simulink model "ChiefMaster_TTC580"  (R2022b)
settings: Solver=FixedStepAuto  StartTime=0.0  StopTime=10  FixedStep=0.01  RelTol=1e-3
values from neighbouring files (symbols this model uses):
  BattBox1_No = single(1)    [Parameters.m]
  BattBox2_No = single(2)    [Parameters.m]
  BattBox3_No = single(3)    [Parameters.m]
  CurrentLB = single(-3)    [Parameters.m]
  CurrentReductionConstant_Lvl0 = single(0.03)    [Parameters.m]
  CurrentReductionConstant_Lvl1 = single(0.05)    [Parameters.m]
  CurrentReductionConstant_Lvl2 = single(0.07)    [Parameters.m]
  CurrentReductionConstant_Lvl3 = single(0.1)    [Parameters.m]
  CurrentUB = single(3)    [Parameters.m]
  DCHV_Minus_In_Delay_ms = single(500)    [Parameters.m]
  FL_sHVC_CellBalanceVoltage_mV = single(3500)    [Parameters.m]
  FL_sInrushCurrent_dividebyzero = single(0.00001)    [Parameters.m]
  FL_u8HMI_BuzzerTimer = uint8(3)    [Parameters.m]
  IP_boActValue = true    [Parameters.m]
  IP_boDeactValue = false    [Parameters.m]
  IP_boInitValue = false    [Parameters.m]
  IP_s_LB = 18000    [Parameters.m]
  IP_s_UB = 22000    [Parameters.m]
  IP_sBatt1_ChargeCurrentMax_Factor = single(0.1)    [Parameters.m]
  IP_sBatt1_ChargeCurrentMax_LB = single(0)    [Parameters.m]
  IP_sBatt1_ChargeCurrentMax_Offset = single(0)    [Parameters.m]
  IP_sBatt1_ChargeCurrentMax_UB = single(6553.5)    [Parameters.m]
  IP_sBatt1_Current_Factor = single(0.1)    [Parameters.m]
  IP_sBatt1_Current_LB = single(-3276.8)    [Parameters.m]
  IP_sBatt1_Current_Offset = single(0)    [Parameters.m]
  IP_sBatt1_Current_UB = single(3276.8)    [Parameters.m]
  IP_sBatt1_DisChargeCurrentMax_Factor = single(0.1)    [Parameters.m]
  IP_sBatt1_DisChargeCurrentMax_LB = single(0)    [Parameters.m]
  IP_sBatt1_DisChargeCurrentMax_Offset = single(0)    [Parameters.m]
  IP_sBatt1_DisChargeCurrentMax_UB = single(6553.5)    [Parameters.m]
  IP_sBatt1_InsulationResistance_Factor = single(5)    [Parameters.m]
  IP_sBatt1_InsulationResistance_LB = single(0)    [Parameters.m]
  IP_sBatt1_InsulationResistance_Offset = single(0)    [Parameters.m]
  IP_sBatt1_InsulationResistance_UB = single(0)    [Parameters.m]
  IP_sBatt1_LiBa_IntResist_mOhm = single(25)    [Parameters.m]
  IP_sBatt1_SOC_Factor = single(1)    [Parameters.m]
  IP_sBatt1_SOC_LB = single(0)    [Parameters.m]
  IP_sBatt1_SOC_Offset = single(0)    [Parameters.m]
  IP_sBatt1_SOC_UB = single(100)    [Parameters.m]
  IP_sBatt1_SOH_Factor = single(1)    [Parameters.m]
  IP_sBatt1_SOH_LB = single(0)    [Parameters.m]
  IP_sBatt1_SOH_Offset = single(0)    [Parameters.m]
  IP_sBatt1_SOH_UB = single(100)    [Parameters.m]
  IP_sBatt1_Ubatt_Factor = single(0.1)    [Parameters.m]
  IP_sBatt1_Ubatt_LB = single(0)    [Parameters.m]
  IP_sBatt1_Ubatt_Offset = single(0)    [Parameters.m]
  IP_sBatt1_Ubatt_UB = single(6553.5)    [Parameters.m]
  IP_sBatt1_UserRi_Factor = single(1)    [Parameters.m]
  IP_sBatt1_UserRi_LB = single(0)    [Parameters.m]
  IP_sBatt1_UserRi_Offset = single(0)    [Parameters.m]
  IP_sBatt1_UserRi_UB = single(255)    [Parameters.m]
  IP_sBatt1_VoltageAtSensor_Factor = single(0.02)    [Parameters.m]
  IP_sBatt1_VoltageAtSensor_LB = single(0)    [Parameters.m]
  IP_sBatt1_VoltageAtSensor_Offset = single(0)    [Parameters.m]
  IP_sBatt1_VoltageAtSensor_UB = single(1310.7)    [Parameters.m]
  IP_sBatt2_LiBa_IntResist_mOhm = single(25)    [Parameters.m]
  IP_sBatt3_LiBa_IntResist_mOhm = single(25)    [Parameters.m]
  IP_sEM_LB = 2000    [Parameters.m]
  IP_sEM_UB = 8000    [Parameters.m]
  IP_sFB_LB = 5000    [Parameters.m]
  IP_sFB_UB = 10000    [Parameters.m]
  IP_sHVIL_LB = 12000    [Parameters.m]
  IP_sHVIL_UB = 15000    [Parameters.m]
  IP_sLoad_Voltage_Factor = single(1)    [Parameters.m]
  IP_sLoad_Voltage_LB = single(0)    [Parameters.m]
  IP_sLoad_Voltage_Offset = single(0)    [Parameters.m]
  IP_sLoad_Voltage_UB = single(65535)    [Parameters.m]
  IP_u8HVIL_Delay_ms = uint8(100)    [Parameters.m]
  IP_u8HW_IN_delay_ms = uint8(100)    [Parameters.m]
  IT_sInsulationSafeValue_kOhm = single(650)    [Parameters.m]
  IT_u8IMD_DelayTime_s = uint8(20)    [Parameters.m]
  MainHV_Minus_In_Delay = single(5)    [Parameters.m]
  MainHV_StatusDelay = single(5)    [Parameters.m]
  NotAvailable_uint16 = single(65535)    [Parameters.m]
  NotAvailable_uint8 = uint8(255)    [Parameters.m]
  OP_boHVIL_Supply = boolean(1)    [Parameters.m]
  SafeCurrentToCloseHV_A = single(5)    [Parameters.m]
  SafeVoltageToCloseHV_V = single(0.5)    [Parameters.m]
  UnexpectedBattChargingFcn_Available = boolean(1)    [Parameters.m]
  Voltage_NA_UB = uint16(65535)    [Parameters.m]
  VoltageSensorAvailableBB1 = boolean(0)    [Parameters.m]
  VoltageSensorAvailableBB2 = boolean(0)    [Parameters.m]
  VoltageSensorAvailableBB3 = boolean(0)    [Parameters.m]
libraries: simulink x184, Library_DataProcessing_v1_1 x167, Library_DataProcessing_v1 x142, libCM x28
(part 1 of 19)
settings Model: TunableVars=SafeCurrentToCloseHV_A,SafeVoltageToCloseHV_V,Voltage_NA_UB,MainHV_Minus_In_Delay,MainHV_StatusDelay,BattBox1_No,BattBox2_No,BattBox3_No,NotAvailable_uint16,NotAvailable_uint8,VoltageSensorAvailableBB1,VoltageSensorAvailableBB2,VoltageSensorAvailableBB3,CurrentLB,CurrentReductionConstant_Lvl0,CurrentReductionConstant_Lvl1,CurrentReductionConstant_Lvl2,CurrentReductionConstant_Lvl3,CurrentUB,FL_sHVC_CellBalanceVoltage_mV,FL_sInrushCurrent_dividebyzero,FL_u8HMI_BuzzerTimer,UnexpectedBattChargingFcn_Available,IT_sInsulationSafeValue_kOhm,DCHV_Minus_In_Delay_ms,IP_u8HW_IN_delay_ms,OP_boHVIL_Supply,IP_u8HVIL_Delay_ms,IT_u8IMD_DelayTime_s  TunableVarsStorageClass=ExportedGlobal,ExportedGlobal,ExportedGlobal,ExportedGlobal,ExportedGlobal,ExportedGlobal,ExportedGlobal,ExportedGlobal,ExportedGlobal,ExportedGlobal,ExportedGlobal,ExportedGlobal,ExportedGlobal,ExportedGlobal,ExportedGlobal,ExportedGlobal,ExportedGlobal,ExportedGlobal,ExportedGlobal,ExportedGlobal,ExportedGlobal,ExportedGlobal,ExportedGlobal,ExportedGlobal,ExportedGlobal,ExportedGlobal,ExportedGlobal,ExportedGlobal,ExportedGlobal  TunableVarsTypeQualifier=,,,,,,,,,,,,,,,,,,,,,,,,,,,,  Creator=SidharthUrbanMobilit  LastModifiedBy=NurdoganUrbanMobilit
settings SolverCC: AlgebraicLoopSolver=TrustRegion
settings OptimizationCC: DefaultUnderspecifiedDataType=single  ZeroExternalMemoryAtStartup=off  ZeroInternalMemoryAtStartup=off  NoFixptDivByZeroProtection=on  EfficientFloat2IntCast=on  EfficientTunableParamExpr=on
settings DebuggingCC: SignalInfNanChecking=error  ParameterPrecisionLossMsg=none  ParameterTunabilityLossMsg=error  UnconnectedInputMsg=warning  UnconnectedOutputMsg=warning  UnconnectedLineMsg=warning  FrameProcessingCompatibilityMsg=none  BusObjectLabelMismatch=error  SFMachineParentedDataDiag=warning
settings ModelReferenceCC: EnableRefExpFcnMdlSchedulingChecks=on
settings SFSimCC: MATLABDynamicMemAlloc=off
settings RTWCC: Description=Embedded Coder  SystemTargetFile=ert.tlc  TemplateMakefile=ert_default_tmf  DLArmComputeVersion=19.05
settings CodeAppCC: ForceParamTrailComments=on  MaxIdLength=100  OperatorAnnotations=on  SimulinkDataObjDesc=on  SFDataObjDesc=on  MATLABFcnDesc=on  CustomSymbolStrFcn=$N$M  CustomSymbolStrFcnArg=$N$M  InsertBlockDesc=on  StateflowObjectComments=on  MATLABSourceComments=on  ReqsInCode=on
settings ERTTargetCC: TargetLangStandard=C99 (ISO)  CodeReplacementLibrary=PLC  GenerateSampleERTMain=on  SupportNonFinite=off  SupportVariableSizeSignals=on  ERTCustomFileTemplate=example_file_process.tlc
settings ConfigComp: PLC_OutputDir=cdsys  PLC_TargetIDE=codesys35  PLC_MultiTBSigbuilderTimeRange=off  PLC_PreserveAliasType=on  PLC_FoldFBCallOutputVar=off  PLC_OverrideDefaultNameLength=on  PLC_InlineEnumCastFunction=off  PLC_RTWMaxIdLength=100  PLC_GenerateReport=off  PLC_LaunchReport=off

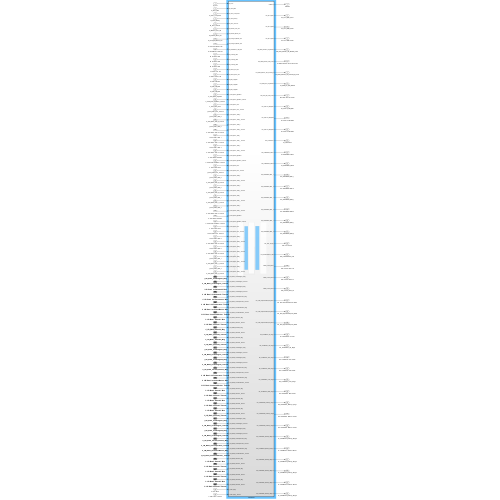
[thumbnail: Simulink's stored preview of the top-level diagram]
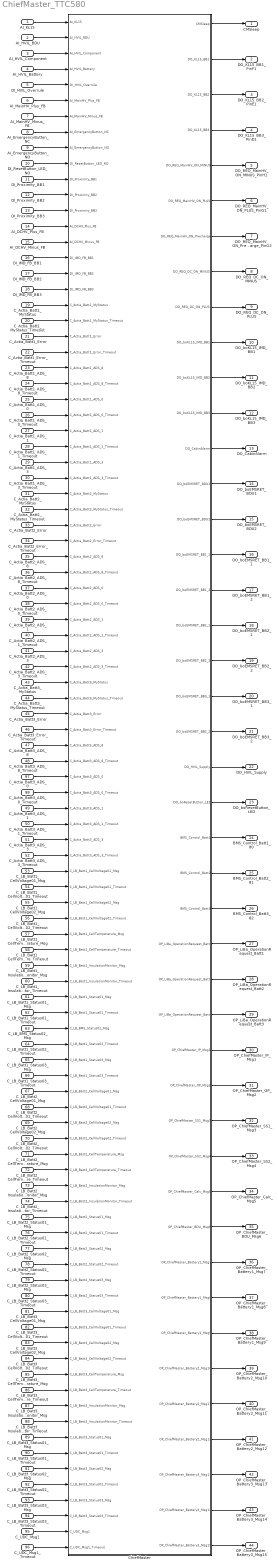
== system ChiefMaster_TTC580 ==
  AI_KL15 : Inport  OutDataTypeStr=single
  AI_HVIL_BDU : Inport  Port=2  OutDataTypeStr=single
  AI_HVIL_Component : Inport  Port=3  OutDataTypeStr=single
  AI_HVIL_Battery : Inport  Port=4  OutDataTypeStr=single
  DI_HVIL_Overrule : Inport  Port=5  OutDataTypeStr=boolean
  AI_MainHV_Plus_FB : Inport  Port=6  OutDataTypeStr=single
  AI_MainHV_Minus_FB : Inport  Port=7  OutDataTypeStr=single
  AI_EmergencyButton_NC : Inport  Port=8  OutDataTypeStr=single
  AI_EmergencyButton_NO : Inport  Port=9  OutDataTypeStr=single
  DI_ResetButton_LED_NO : Inport  Port=10  OutDataTypeStr=boolean
  DI_Proximity_BB1 : Inport  Port=11  OutDataTypeStr=boolean
  DI_Proximity_BB2 : Inport  Port=12  OutDataTypeStr=boolean
  DI_Proximity_BB3 : Inport  Port=13  OutDataTypeStr=boolean
  AI_DCHV_Plus_FB : Inport  Port=14  OutDataTypeStr=single
  AI_DCHV_Minus_FB : Inport  Port=15  OutDataTypeStr=single
  DI_IMD_FB_BB1 : Inport  Port=16
  DI_IMD_FB_BB2 : Inport  Port=17
  DI_IMD_FB_BB3 : Inport  Port=18
  C_Actia_Batt1_MyStatus : Inport  Port=19  OutDataTypeStr=uint8
  C_Actia_Batt1_MyStatus_Timeout : Inport  Port=20  OutDataTypeStr=boolean
  C_Actia_Batt1_Error : Inport  Port=21  OutDataTypeStr=uint8
  C_Actia_Batt1_Error_Timeout : Inport  Port=22  OutDataTypeStr=boolean
  C_Actia_Batt1_ADS_8 : Inport  Port=23  OutDataTypeStr=uint8
  C_Actia_Batt1_ADS_8_Timeout : Inport  Port=24  OutDataTypeStr=boolean
  C_Actia_Batt1_ADS_0 : Inport  Port=25
  C_Actia_Batt1_ADS_0_Timeout : Inport  Port=26
  C_Actia_Batt1_ADS_1 : Inport  Port=27  OutDataTypeStr=uint8
  C_Actia_Batt1_ADS_1_Timeout : Inport  Port=28  OutDataTypeStr=boolean
  C_Actia_Batt1_ADS_3 : Inport  Port=29  OutDataTypeStr=uint8
  C_Actia_Batt1_ADS_3_Timeout : Inport  Port=30  OutDataTypeStr=boolean
  C_Actia_Batt2_MyStatus : Inport  Port=31  OutDataTypeStr=uint8
  C_Actia_Batt2_MyStatus_Timeout : Inport  Port=32  OutDataTypeStr=boolean
  C_Actia_Batt2_Error : Inport  Port=33  OutDataTypeStr=uint8
  C_Actia_Batt2_Error_Timeout : Inport  Port=34  OutDataTypeStr=boolean
  C_Actia_Batt2_ADS_8 : Inport  Port=35  OutDataTypeStr=uint8
  C_Actia_Batt2_ADS_8_Timeout : Inport  Port=36  OutDataTypeStr=boolean
  C_Actia_Batt2_ADS_0 : Inport  Port=37
  C_Actia_Batt2_ADS_0_Timeout : Inport  Port=38
  C_Actia_Batt2_ADS_1 : Inport  Port=39  OutDataTypeStr=uint8
  C_Actia_Batt2_ADS_1_Timeout : Inport  Port=40  OutDataTypeStr=boolean
  C_Actia_Batt2_ADS_3 : Inport  Port=41  OutDataTypeStr=uint8
  C_Actia_Batt2_ADS_3_Timeout : Inport  Port=42  OutDataTypeStr=boolean
  C_Actia_Batt3_MyStatus : Inport  Port=43  OutDataTypeStr=uint8
  C_Actia_Batt3_MyStatus_Timeout : Inport  Port=44  OutDataTypeStr=boolean
  C_Actia_Batt3_Error : Inport  Port=45  OutDataTypeStr=uint8
  C_Actia_Batt3_Error_Timeout : Inport  Port=46  OutDataTypeStr=boolean
  C_Actia_Batt3_ADS_8 : Inport  Port=47  OutDataTypeStr=uint8
  C_Actia_Batt3_ADS_8_Timeout : Inport  Port=48  OutDataTypeStr=boolean
  C_Actia_Batt3_ADS_1 : Inport  Port=49  OutDataTypeStr=uint8
  C_Actia_Batt3_ADS_1_Timeout : Inport  Port=50  OutDataTypeStr=boolean
  C_Actia_Batt3_ADS_3 : Inport  Port=51  OutDataTypeStr=uint8
  C_Actia_Batt3_ADS_3_Timeout : Inport  Port=52  OutDataTypeStr=boolean
  C_LB_Batt1_CellVoltage01_Msg : Inport  Port=53  OutDataTypeStr=uint8
  C_LB_Batt1_CellVoltage01_Timeout : Inport  Port=54  OutDataTypeStr=boolean
  C_LB_Batt1_CellVoltage02_Msg : Inport  Port=55  OutDataTypeStr=uint8
  C_LB_Batt1_CellVoltage02_Timeout : Inport  Port=56  OutDataTypeStr=boolean
  C_LB_Batt1_CellTemperature_Msg : Inport  Port=57  OutDataTypeStr=uint8
  C_LB_Batt1_CellTemperature_Timeout : Inport  Port=58  OutDataTypeStr=boolean
  C_LB_Batt1_InsulationMonitor_Msg : Inport  Port=59  OutDataTypeStr=uint8
  C_LB_Batt1_InsulationMonitor_Timeout : Inport  Port=60
  C_LB_Batt1_Status01_Msg : Inport  Port=61
  C_LB_Batt1_Status01_Timeout : Inport  Port=62
  C_LB_BMS_Status02_Msg : Inport  Port=63
  C_LB_Batt1_Status02_Timeout : Inport  Port=64
  C_LB_Batt1_Status03_Msg : Inport  Port=65
  C_LB_Batt1_Status03_Timeout : Inport  Port=66
  C_LB_Batt2_CellVoltage01_Msg : Inport  Port=67
  C_LB_Batt2_CellVoltage01_Timeout : Inport  Port=68
  C_LB_Batt2_CellVoltage02_Msg : Inport  Port=69  OutDataTypeStr=uint8
  C_LB_Batt2_CellVoltage02_Timeout : Inport  Port=70
  C_LB_Batt2_CellTemperature_Msg : Inport  Port=71  OutDataTypeStr=uint8
  C_LB_Batt2_CellTemperature_Timeout : Inport  Port=72
  C_LB_Batt2_InsulationMonitor_Msg : Inport  Port=73  OutDataTypeStr=uint8
  C_LB_Batt2_InsulationMonitor_Timeout : Inport  Port=74
  C_LB_Batt2_Status01_Msg : Inport  Port=75  OutDataTypeStr=uint8
  C_LB_Batt2_Status01_Timeout : Inport  Port=76
  C_LB_Batt2_Status02_Msg : Inport  Port=77  OutDataTypeStr=uint8
  C_LB_Batt2_Status02_Timeout : Inport  Port=78
  C_LB_Batt2_Status03_Msg : Inport  Port=79  OutDataTypeStr=uint8
  C_LB_Batt2_Status03_Timeout : Inport  Port=80
  C_LB_Batt3_CellVoltage01_Msg : Inport  Port=81  OutDataTypeStr=uint8
  C_LB_Batt3_CellVoltage01_Timeout : Inport  Port=82
  C_LB_Batt3_CellVoltage02_Msg : Inport  Port=83  OutDataTypeStr=uint8
  C_LB_Batt3_CellVoltage02_Timeout : Inport  Port=84
  C_LB_Batt3_CellTemperature_Msg : Inport  Port=85  OutDataTypeStr=uint8
  C_LB_Batt3_CellTemperature_Timeout : Inport  Port=86
  C_LB_Batt3_InsulationMonitor_Msg : Inport  Port=87  OutDataTypeStr=uint8
  C_LB_Batt3_InsulationMonitor_Timeout : Inport  Port=88
  C_LB_Batt3_Status01_Msg : Inport  Port=89  OutDataTypeStr=uint8
  C_LB_Batt3_Status01_Timeout : Inport  Port=90
  C_LB_Batt3_Status02_Msg : Inport  Port=91  OutDataTypeStr=uint8
  C_LB_Batt3_Status02_Timeout : Inport  Port=92
  C_LB_Batt3_Status03_Msg : Inport  Port=93  OutDataTypeStr=uint8
  C_LB_Batt3_Status03_Timeout : Inport  Port=94
  C_UDC_Msg1 : Inport  Port=95  OutDataTypeStr=uint8
  C_UDC_Msg1_Timeout : Inport  Port=96
  C_Actia_Batt3_ADS_0 : Inport  Port=97
  C_Actia_Batt3_ADS_0_Timeout : Inport  Port=98
  ChiefMaster : Subsystem  TreatAsAtomicUnit=on
  CMSleep : Outport
  DO_KL15_BB1_PinF1 : Outport  Port=2
  DO_KL15_BB2_PinE1 : Outport  Port=3
  DO_KL15_BB3_PinD1 : Outport  Port=4
  DO_REQ_MainHV_ON_MINUS_PinH1 : Outport  Port=5
  DO_REQ_MainHV_ON_PLUS_PinG1 : Outport  Port=6
  DO_REQ_MainHV_ON_Precharge_PinG2 : Outport  Port=7
  DO_REQ_DC_ON_MINUS : Outport  Port=8
  DO_REQ_DC_ON_PLUS : Outport  Port=9
  DO_boKL15_IMD_BB1 : Outport  Port=10
  DO_boKL15_IMD_BB2 : Outport  Port=11
  DO_boKL15_IMD_BB3 : Outport  Port=12
  DO_CabinAlarm : Outport  Port=13
  DO_boEMSRET_BDU1 : Outport  Port=14  OutDataTypeStr=boolean
  DO_boEMSRET_BDU2 : Outport  Port=15  OutDataTypeStr=boolean
  DO_boEMSRET_BB1_1 : Outport  Port=16  OutDataTypeStr=boolean
  DO_boEMSRET_BB1_2 : Outport  Port=17  OutDataTypeStr=boolean
  DO_boEMSRET_BB2_1 : Outport  Port=18  OutDataTypeStr=boolean
  DO_boEMSRET_BB2_2 : Outport  Port=19  OutDataTypeStr=boolean
  DO_boEMSRET_BB3_1 : Outport  Port=20  OutDataTypeStr=boolean
  DO_boEMSRET_BB3_2 : Outport  Port=21  OutDataTypeStr=boolean
  DO_HVIL_Supply : Outport  Port=22  OutDataTypeStr=boolean
  DO_boResetButton_LED : Outport  Port=23  OutDataTypeStr=boolean
  BMS_Control_Batt1_80 : Outport  Port=24
  BMS_Control_Batt2_81 : Outport  Port=25
  BMS_Control_Batt3_82 : Outport  Port=26
  OP_LiBa_OperationRequest_Batt1 : Outport  Port=27
  OP_LiBa_OperationRequest_Batt2 : Outport  Port=28
  OP_LiBa_OperationRequest_Batt3 : Outport  Port=29
  OP_ChiefMaster_IP_Msg1 : Outport  Port=30
  OP_ChiefMaster_OP_Msg2 : Outport  Port=31
  OP_ChiefMaster_SS1_Msg3 : Outport  Port=32
  OP_ChiefMaster_SS2_Msg4 : Outport  Port=33
  OP_ChiefMaster_Calc_Msg5 : Outport  Port=34
  OP_ChiefMaster_BDU_Msg6 : Outport  Port=35
  OP_ChiefMaster_Battery1_Msg7 : Outport  Port=36
  OP_ChiefMaster_Battery1_Msg8 : Outport  Port=37
  OP_ChiefMaster_Battery1_Msg9 : Outport  Port=38
  OP_ChiefMaster_Battery2_Msg10 : Outport  Port=39
  OP_ChiefMaster_Battery2_Msg11 : Outport  Port=40
  OP_ChiefMaster_Battery2_Msg12 : Outport  Port=41
  OP_ChiefMaster_Battery3_Msg13 : Outport  Port=42
  OP_ChiefMaster_Battery3_Msg14 : Outport  Port=43
  OP_ChiefMaster_Battery3_Msg15 : Outport  Port=44
  wires:
  C_LB_Batt1_Status03_Timeout/1 -> ChiefMaster/68(C_LB_Batt1_Status03_Timeout)
  ChiefMaster/2(DO_KL15_BB1) -> DO_KL15_BB1_PinF1/1
  C_UDC_Msg1_Timeout/1 -> ChiefMaster/98(C_UDC_Msg1_Timeout)
  ChiefMaster/26(BMS_Control_Batt3) -> BMS_Control_Batt3_82/1
  ChiefMaster/24(BMS_Control_Batt1) -> BMS_Control_Batt1_80/1
  ChiefMaster/6(DO_REQ_MainHV_ON_PLUS) -> DO_REQ_MainHV_ON_PLUS_PinG1/1
  ChiefMaster/4(DO_KL15_BB3) -> DO_KL15_BB3_PinD1/1
  ChiefMaster/3(DO_KL15_BB2) -> DO_KL15_BB2_PinE1/1
  ChiefMaster/1(CMSleep) -> CMSleep/1
  C_LB_Batt1_Status01_Msg/1 -> ChiefMaster/63(C_LB_Batt1_Status01_Msg)
  C_LB_Batt1_CellVoltage01_Msg/1 -> ChiefMaster/55(C_LB_Batt1_CellVoltage01_Msg)
  C_LB_Batt1_InsulationMonitor_Msg/1 -> ChiefMaster/61(C_LB_Batt1_InsulationMonitor_Msg)
  C_LB_Batt1_CellTemperature_Timeout/1 -> ChiefMaster/60(C_LB_Batt1_CellTemperature_Timeout)
  C_LB_Batt1_Status02_Timeout/1 -> ChiefMaster/66(C_LB_Batt1_Status02_Timeout)
  C_LB_Batt1_CellVoltage02_Timeout/1 -> ChiefMaster/58(C_LB_Batt1_CellVoltage02_Timeout)
  C_LB_Batt1_Status01_Timeout/1 -> ChiefMaster/64(C_LB_Batt1_Status01_Timeout)
  C_LB_Batt1_CellVoltage01_Timeout/1 -> ChiefMaster/56(C_LB_Batt1_CellVoltage01_Timeout)
  C_LB_Batt1_CellVoltage02_Msg/1 -> ChiefMaster/57(C_LB_Batt1_CellVoltage02_Msg)
  C_LB_Batt1_Status03_Msg/1 -> ChiefMaster/67(C_LB_Batt1_Status03_Msg)
  C_LB_Batt1_CellTemperature_Msg/1 -> ChiefMaster/59(C_LB_Batt1_CellTemperature_Msg)
  C_LB_Batt1_InsulationMonitor_Timeout/1 -> ChiefMaster/62(C_LB_Batt1_InsulationMonitor_Timeout)
  C_LB_BMS_Status02_Msg/1 -> ChiefMaster/65(C_LB_BMS_Status02_Msg)
  C_UDC_Msg1/1 -> ChiefMaster/97(C_UDC_Msg1)
  ChiefMaster/25(BMS_Control_Batt2) -> BMS_Control_Batt2_81/1
  ChiefMaster/7(DO_REQ_MainHV_ON_Precharge) -> DO_REQ_MainHV_ON_Precharge_PinG2/1
  ChiefMaster/5(DO_REQ_MainHV_ON_MINUS) -> DO_REQ_MainHV_ON_MINUS_PinH1/1
  C_LB_Batt3_CellVoltage01_Timeout/1 -> ChiefMaster/84(C_LB_Batt3_CellVoltage01_Timeout)
  C_LB_Batt3_CellVoltage02_Msg/1 -> ChiefMaster/85(C_LB_Batt3_CellVoltage02_Msg)
  C_LB_Batt2_CellTemperature_Msg/1 -> ChiefMaster/73(C_LB_Batt2_CellTemperature_Msg)
  C_LB_Batt2_CellVoltage02_Msg/1 -> ChiefMaster/71(C_LB_Batt2_CellVoltage02_Msg)
  C_LB_Batt2_CellVoltage02_Timeout/1 -> ChiefMaster/72(C_LB_Batt2_CellVoltage02_Timeout)
  C_LB_Batt2_CellTemperature_Timeout/1 -> ChiefMaster/74(C_LB_Batt2_CellTemperature_Timeout)
  C_LB_Batt3_CellVoltage02_Timeout/1 -> ChiefMaster/86(C_LB_Batt3_CellVoltage02_Timeout)
  C_LB_Batt3_CellTemperature_Msg/1 -> ChiefMaster/87(C_LB_Batt3_CellTemperature_Msg)
  C_LB_Batt3_CellTemperature_Timeout/1 -> ChiefMaster/88(C_LB_Batt3_CellTemperature_Timeout)
  C_LB_Batt3_CellVoltage01_Msg/1 -> ChiefMaster/83(C_LB_Batt3_CellVoltage01_Msg)
  C_LB_Batt3_InsulationMonitor_Msg/1 -> ChiefMaster/89(C_LB_Batt3_InsulationMonitor_Msg)
  C_LB_Batt3_InsulationMonitor_Timeout/1 -> ChiefMaster/90(C_LB_Batt3_InsulationMonitor_Timeout)
  C_LB_Batt2_CellVoltage01_Timeout/1 -> ChiefMaster/70(C_LB_Batt2_CellVoltage01_Timeout)
  C_LB_Batt3_Status01_Msg/1 -> ChiefMaster/91(C_LB_Batt3_Status01_Msg)
  C_LB_Batt3_Status01_Timeout/1 -> ChiefMaster/92(C_LB_Batt3_Status01_Timeout)
  C_LB_Batt3_Status02_Msg/1 -> ChiefMaster/93(C_LB_Batt3_Status02_Msg)
  C_LB_Batt3_Status02_Timeout/1 -> ChiefMaster/94(C_LB_Batt3_Status02_Timeout)
  C_LB_Batt3_Status03_Msg/1 -> ChiefMaster/95(C_LB_Batt3_Status03_Msg)
  C_LB_Batt3_Status03_Timeout/1 -> ChiefMaster/96(C_LB_Batt3_Status03_Timeout)
  C_LB_Batt2_CellVoltage01_Msg/1 -> ChiefMaster/69(C_LB_Batt2_CellVoltage01_Msg)
  C_LB_Batt2_InsulationMonitor_Msg/1 -> ChiefMaster/75(C_LB_Batt2_InsulationMonitor_Msg)
  C_LB_Batt2_InsulationMonitor_Timeout/1 -> ChiefMaster/76(C_LB_Batt2_InsulationMonitor_Timeout)
  C_LB_Batt2_Status01_Msg/1 -> ChiefMaster/77(C_LB_Batt2_Status01_Msg)
  C_LB_Batt2_Status01_Timeout/1 -> ChiefMaster/78(C_LB_Batt2_Status01_Timeout)
  C_LB_Batt2_Status02_Msg/1 -> ChiefMaster/79(C_LB_Batt2_Status02_Msg)
  C_LB_Batt2_Status02_Timeout/1 -> ChiefMaster/80(C_LB_Batt2_Status02_Timeout)
  C_LB_Batt2_Status03_Msg/1 -> ChiefMaster/81(C_LB_Batt2_Status03_Msg)
  C_LB_Batt2_Status03_Timeout/1 -> ChiefMaster/82(C_LB_Batt2_Status03_Timeout)
  ChiefMaster/28(OP_LiBa_OperationRequest_Batt2) -> OP_LiBa_OperationRequest_Batt2/1
  ChiefMaster/29(OP_LiBa_OperationRequest_Batt3) -> OP_LiBa_OperationRequest_Batt3/1
  ChiefMaster/27(OP_LiBa_OperationRequest_Batt1) -> OP_LiBa_OperationRequest_Batt1/1
  DI_Proximity_BB1/1 -> ChiefMaster/11(DI_Proximity_BB1)
  AI_HVIL_Component/1 -> ChiefMaster/3(AI_HVIL_Component)
  AI_HVIL_BDU/1 -> ChiefMaster/2(AI_HVIL_BDU)
  AI_EmergencyButton_NO/1 -> ChiefMaster/9(AI_EmergencyButton_NO)
  AI_HVIL_Battery/1 -> ChiefMaster/4(AI_HVIL_Battery)
  DI_Proximity_BB3/1 -> ChiefMaster/13(DI_Proximity_BB3)
  AI_DCHV_Plus_FB/1 -> ChiefMaster/14(AI_DCHV_Plus_FB)
  AI_KL15/1 -> ChiefMaster/1(AI_KL15)
  AI_MainHV_Minus_FB/1 -> ChiefMaster/7(AI_MainHV_Minus_FB)
  DI_Proximity_BB2/1 -> ChiefMaster/12(DI_Proximity_BB2)
  AI_EmergencyButton_NC/1 -> ChiefMaster/8(AI_EmergencyButton_NC)
  AI_DCHV_Minus_FB/1 -> ChiefMaster/15(AI_DCHV_Minus_FB)
  DI_ResetButton_LED_NO/1 -> ChiefMaster/10(DI_ResetButton_LED_NO)
  AI_MainHV_Plus_FB/1 -> ChiefMaster/6(AI_MainHV_Plus_FB)
  C_Actia_Batt1_ADS_3/1 -> ChiefMaster/29(C_Actia_Batt1_ADS_3)
  C_Actia_Batt1_ADS_1/1 -> ChiefMaster/27(C_Actia_Batt1_ADS_1)
  C_Actia_Batt1_ADS_8_Timeout/1 -> ChiefMaster/24(C_Actia_Batt1_ADS_8_Timeout)
  C_Actia_Batt3_MyStatus/1 -> ChiefMaster/43(C_Actia_Batt3_MyStatus)
  C_Actia_Batt2_ADS_3_Timeout/1 -> ChiefMaster/42(C_Actia_Batt2_ADS_3_Timeout)
  C_Actia_Batt3_ADS_3_Timeout/1 -> ChiefMaster/54(C_Actia_Batt3_ADS_3_Timeout)
  C_Actia_Batt3_MyStatus_Timeout/1 -> ChiefMaster/44(C_Actia_Batt3_MyStatus_Timeout)
  C_Actia_Batt2_Error/1 -> ChiefMaster/33(C_Actia_Batt2_Error)
  C_Actia_Batt2_ADS_3/1 -> ChiefMaster/41(C_Actia_Batt2_ADS_3)
  C_Actia_Batt3_Error/1 -> ChiefMaster/45(C_Actia_Batt3_Error)
  C_Actia_Batt1_MyStatus/1 -> ChiefMaster/19(C_Actia_Batt1_MyStatus)
  C_Actia_Batt1_Error/1 -> ChiefMaster/21(C_Actia_Batt1_Error)
  C_Actia_Batt2_Error_Timeout/1 -> ChiefMaster/34(C_Actia_Batt2_Error_Timeout)
  C_Actia_Batt1_ADS_8/1 -> ChiefMaster/23(C_Actia_Batt1_ADS_8)
  C_Actia_Batt3_ADS_1/1 -> ChiefMaster/51(C_Actia_Batt3_ADS_1)
  C_Actia_Batt3_ADS_3/1 -> ChiefMaster/53(C_Actia_Batt3_ADS_3)
  C_Actia_Batt3_ADS_8_Timeout/1 -> ChiefMaster/48(C_Actia_Batt3_ADS_8_Timeout)
  C_Actia_Batt1_MyStatus_Timeout/1 -> ChiefMaster/20(C_Actia_Batt1_MyStatus_Timeout)
  C_Actia_Batt3_Error_Timeout/1 -> ChiefMaster/46(C_Actia_Batt3_Error_Timeout)
  C_Actia_Batt3_ADS_8/1 -> ChiefMaster/47(C_Actia_Batt3_ADS_8)
  C_Actia_Batt2_MyStatus/1 -> ChiefMaster/31(C_Actia_Batt2_MyStatus)
  C_Actia_Batt2_MyStatus_Timeout/1 -> ChiefMaster/32(C_Actia_Batt2_MyStatus_Timeout)
  C_Actia_Batt2_ADS_8/1 -> ChiefMaster/35(C_Actia_Batt2_ADS_8)
  C_Actia_Batt1_Error_Timeout/1 -> ChiefMaster/22(C_Actia_Batt1_Error_Timeout)
  C_Actia_Batt2_ADS_8_Timeout/1 -> ChiefMaster/36(C_Actia_Batt2_ADS_8_Timeout)
  C_Actia_Batt3_ADS_1_Timeout/1 -> ChiefMaster/52(C_Actia_Batt3_ADS_1_Timeout)
  C_Actia_Batt2_ADS_1/1 -> ChiefMaster/39(C_Actia_Batt2_ADS_1)
  C_Actia_Batt2_ADS_1_Timeout/1 -> ChiefMaster/40(C_Actia_Batt2_ADS_1_Timeout)
  C_Actia_Batt1_ADS_1_Timeout/1 -> ChiefMaster/28(C_Actia_Batt1_ADS_1_Timeout)
  C_Actia_Batt1_ADS_3_Timeout/1 -> ChiefMaster/30(C_Actia_Batt1_ADS_3_Timeout)
  ChiefMaster/43(OP_ChiefMaster_Battery3_Msg14) -> OP_ChiefMaster_Battery3_Msg14/1
  ChiefMaster/42(OP_ChiefMaster_Battery3_Msg13) -> OP_ChiefMaster_Battery3_Msg13/1
  ChiefMaster/30(OP_ChiefMaster_IP_Msg1) -> OP_ChiefMaster_IP_Msg1/1
  ChiefMaster/40(OP_ChiefMaster_Battery2_Msg11) -> OP_ChiefMaster_Battery2_Msg11/1
  ChiefMaster/31(OP_ChiefMaster_OP_Msg2) -> OP_ChiefMaster_OP_Msg2/1
  ChiefMaster/32(OP_ChiefMaster_SS1_Msg3) -> OP_ChiefMaster_SS1_Msg3/1
  ChiefMaster/33(OP_ChiefMaster_SS2_Msg4) -> OP_ChiefMaster_SS2_Msg4/1
  ChiefMaster/35(OP_ChiefMaster_BDU_Msg6) -> OP_ChiefMaster_BDU_Msg6/1
  ChiefMaster/34(OP_ChiefMaster_Calc_Msg5) -> OP_ChiefMaster_Calc_Msg5/1
  ChiefMaster/36(OP_ChiefMaster_Battery1_Msg7) -> OP_ChiefMaster_Battery1_Msg7/1
  ChiefMaster/37(OP_ChiefMaster_Battery1_Msg8) -> OP_ChiefMaster_Battery1_Msg8/1
  ChiefMaster/39(OP_ChiefMaster_Battery2_Msg10) -> OP_ChiefMaster_Battery2_Msg10/1
  ChiefMaster/8(DO_REQ_DC_ON_MINUS) -> DO_REQ_DC_ON_MINUS/1
  ChiefMaster/9(DO_REQ_DC_ON_PLUS) -> DO_REQ_DC_ON_PLUS/1
  C_Actia_Batt1_ADS_0/1 -> ChiefMaster/25(C_Actia_Batt1_ADS_0)
  C_Actia_Batt1_ADS_0_Timeout/1 -> ChiefMaster/26(C_Actia_Batt1_ADS_0_Timeout)
  C_Actia_Batt2_ADS_0/1 -> ChiefMaster/37(C_Actia_Batt2_ADS_0)
  C_Actia_Batt2_ADS_0_Timeout/1 -> ChiefMaster/38(C_Actia_Batt2_ADS_0_Timeout)
  C_Actia_Batt3_ADS_0_Timeout/1 -> ChiefMaster/50(C_Actia_Batt3_ADS_0_Timeout)
  C_Actia_Batt3_ADS_0/1 -> ChiefMaster/49(C_Actia_Batt3_ADS_0)
  ChiefMaster/38(OP_ChiefMaster_Battery1_Msg9) -> OP_ChiefMaster_Battery1_Msg9/1
  ChiefMaster/41(OP_ChiefMaster_Battery2_Msg12) -> OP_ChiefMaster_Battery2_Msg12/1
  ChiefMaster/44(OP_ChiefMaster_Battery3_Msg15) -> OP_ChiefMaster_Battery3_Msg15/1
  DI_HVIL_Overrule/1 -> ChiefMaster/5(DI_HVIL_Overrule)
  ChiefMaster/10(DO_boKL15_IMD_BB1) -> DO_boKL15_IMD_BB1/1
  ChiefMaster/11(DO_boKL15_IMD_BB2) -> DO_boKL15_IMD_BB2/1
  ChiefMaster/12(DO_boKL15_IMD_BB3) -> DO_boKL15_IMD_BB3/1
  DI_IMD_FB_BB1/1 -> ChiefMaster/16(DI_IMD_FB_BB1)
  DI_IMD_FB_BB2/1 -> ChiefMaster/17(DI_IMD_FB_BB2)
  DI_IMD_FB_BB3/1 -> ChiefMaster/18(DI_IMD_FB_BB3)
  ChiefMaster/13(DO_CabinAlarm) -> DO_CabinAlarm/1
  ChiefMaster/14(DO_boEMSRET_BDU1) -> DO_boEMSRET_BDU1/1
  ChiefMaster/15(DO_boEMSRET_BDU2) -> DO_boEMSRET_BDU2/1
  ChiefMaster/16(DO_boEMSRET_BB1_1) -> DO_boEMSRET_BB1_1/1
  ChiefMaster/17(DO_boEMSRET_BB1_2) -> DO_boEMSRET_BB1_2/1
  ChiefMaster/18(DO_boEMSRET_BB2_1) -> DO_boEMSRET_BB2_1/1
  ChiefMaster/19(DO_boEMSRET_BB2_2) -> DO_boEMSRET_BB2_2/1
  ChiefMaster/20(DO_boEMSRET_BB3_1) -> DO_boEMSRET_BB3_1/1
  ChiefMaster/21(DO_boEMSRET_BB3_2) -> DO_boEMSRET_BB3_2/1
  ChiefMaster/22(DO_HVIL_Supply) -> DO_HVIL_Supply/1
  ChiefMaster/23(DO_boResetButton_LED) -> DO_boResetButton_LED/1

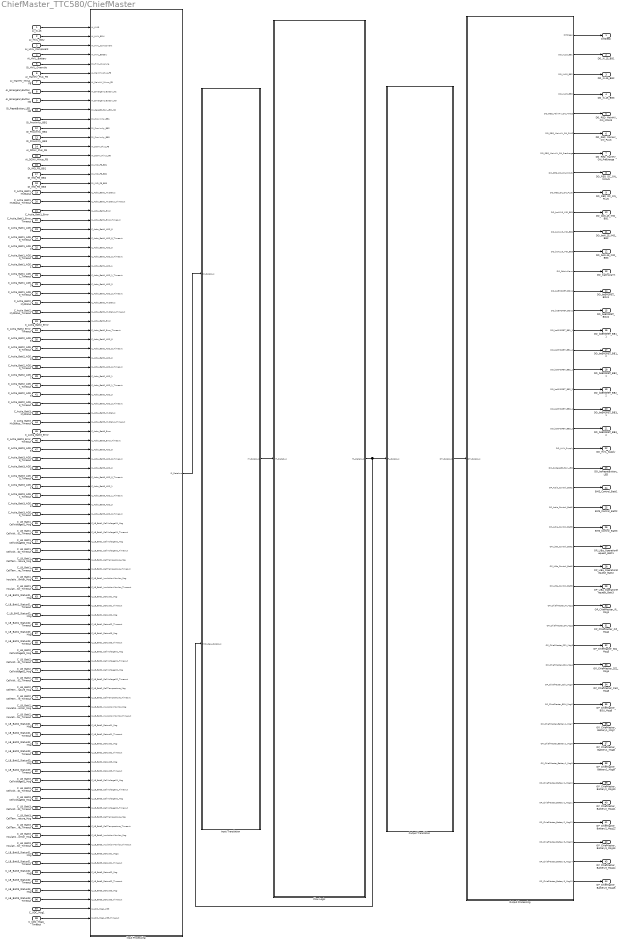
== system ChiefMaster_TTC580/ChiefMaster ==
  AI_KL15 : Inport  OutDataTypeStr=single
  AI_HVIL_BDU : Inport  Port=2  OutDataTypeStr=single
  AI_HVIL_Component : Inport  Port=3  OutDataTypeStr=single
  AI_HVIL_Battery : Inport  Port=4  OutDataTypeStr=single
  DI_HVIL_Overrule : Inport  Port=5  OutDataTypeStr=boolean
  AI_MainHV_Plus_FB : Inport  Port=6  OutDataTypeStr=single
  AI_MainHV_Minus_FB : Inport  Port=7  OutDataTypeStr=single
  AI_EmergencyButton_NC : Inport  Port=8  OutDataTypeStr=single
  AI_EmergencyButton_NO : Inport  Port=9
  DI_ResetButton_LED_NO : Inport  Port=10
  DI_Proximity_BB1 : Inport  Port=11
  DI_Proximity_BB2 : Inport  Port=12
  DI_Proximity_BB3 : Inport  Port=13
  AI_DCHV_Plus_FB : Inport  Port=14  OutDataTypeStr=single
  AI_DCHV_Minus_FB : Inport  Port=15  OutDataTypeStr=single
  DI_IMD_FB_BB1 : Inport  Port=16  OutDataTypeStr=boolean
  DI_IMD_FB_BB2 : Inport  Port=17  OutDataTypeStr=boolean
  DI_IMD_FB_BB3 : Inport  Port=18  OutDataTypeStr=boolean
  C_Actia_Batt1_MyStatus : Inport  Port=19  OutDataTypeStr=uint8
  C_Actia_Batt1_MyStatus_Timeout : Inport  Port=20  OutDataTypeStr=boolean
  C_Actia_Batt1_Error : Inport  Port=21  OutDataTypeStr=uint8
  C_Actia_Batt1_Error_Timeout : Inport  Port=22  OutDataTypeStr=boolean
  C_Actia_Batt1_ADS_8 : Inport  Port=23  OutDataTypeStr=uint8
  C_Actia_Batt1_ADS_8_Timeout : Inport  Port=24  OutDataTypeStr=boolean
  C_Actia_Batt1_ADS_0 : Inport  Port=25
  C_Actia_Batt1_ADS_0_Timeout : Inport  Port=26
  C_Actia_Batt1_ADS_1 : Inport  Port=27  OutDataTypeStr=uint8
  C_Actia_Batt1_ADS_1_Timeout : Inport  Port=28  OutDataTypeStr=boolean
  C_Actia_Batt1_ADS_3 : Inport  Port=29  OutDataTypeStr=uint8
  C_Actia_Batt1_ADS_3_Timeout : Inport  Port=30  OutDataTypeStr=boolean
  C_Actia_Batt2_MyStatus : Inport  Port=31  OutDataTypeStr=uint8
  C_Actia_Batt2_MyStatus_Timeout : Inport  Port=32  OutDataTypeStr=boolean
  C_Actia_Batt2_Error : Inport  Port=33  OutDataTypeStr=uint8
  C_Actia_Batt2_Error_Timeout : Inport  Port=34  OutDataTypeStr=boolean
  C_Actia_Batt2_ADS_8 : Inport  Port=35  OutDataTypeStr=uint8
  C_Actia_Batt2_ADS_8_Timeout : Inport  Port=36  OutDataTypeStr=boolean
  C_Actia_Batt2_ADS_0 : Inport  Port=37
  C_Actia_Batt2_ADS_0_Timeout : Inport  Port=38
  C_Actia_Batt2_ADS_1 : Inport  Port=39  OutDataTypeStr=uint8
  C_Actia_Batt2_ADS_1_Timeout : Inport  Port=40  OutDataTypeStr=boolean
  C_Actia_Batt2_ADS_3 : Inport  Port=41  OutDataTypeStr=uint8
  C_Actia_Batt2_ADS_3_Timeout : Inport  Port=42  OutDataTypeStr=boolean
  C_Actia_Batt3_MyStatus : Inport  Port=43  OutDataTypeStr=uint8
  C_Actia_Batt3_MyStatus_Timeout : Inport  Port=44  OutDataTypeStr=boolean
  C_Actia_Batt3_Error : Inport  Port=45  OutDataTypeStr=uint8
  C_Actia_Batt3_Error_Timeout : Inport  Port=46  OutDataTypeStr=boolean
  C_Actia_Batt3_ADS_8 : Inport  Port=47  OutDataTypeStr=uint8
  C_Actia_Batt3_ADS_8_Timeout : Inport  Port=48  OutDataTypeStr=boolean
  C_Actia_Batt3_ADS_0 : Inport  Port=49
  C_Actia_Batt3_ADS_0_Timeout : Inport  Port=50
  C_Actia_Batt3_ADS_1 : Inport  Port=51  OutDataTypeStr=uint8
  C_Actia_Batt3_ADS_1_Timeout : Inport  Port=52  OutDataTypeStr=boolean
  C_Actia_Batt3_ADS_3 : Inport  Port=53  OutDataTypeStr=uint8
  C_Actia_Batt3_ADS_3_Timeout : Inport  Port=54  OutDataTypeStr=boolean
  C_LB_Batt1_CellVoltage01_Msg : Inport  Port=55
  C_LB_Batt1_CellVoltage01_Timeout : Inport  Port=56
  C_LB_Batt1_CellVoltage02_Msg : Inport  Port=57
  C_LB_Batt1_CellVoltage02_Timeout : Inport  Port=58
  C_LB_Batt1_CellTemperature_Msg : Inport  Port=59
  C_LB_Batt1_CellTemperature_Timeout : Inport  Port=60
  C_LB_Batt1_InsulationMonitor_Msg : Inport  Port=61
  C_LB_Batt1_InsulationMonitor_Timeout : Inport  Port=62
  C_LB_Batt1_Status01_Msg : Inport  Port=63
  C_LB_Batt1_Status01_Timeout : Inport  Port=64
  C_LB_BMS_Status02_Msg : Inport  Port=65
  C_LB_Batt1_Status02_Timeout : Inport  Port=66
  C_LB_Batt1_Status03_Msg : Inport  Port=67
  C_LB_Batt1_Status03_Timeout : Inport  Port=68
  C_LB_Batt2_CellVoltage01_Msg : Inport  Port=69
  C_LB_Batt2_CellVoltage01_Timeout : Inport  Port=70
  C_LB_Batt2_CellVoltage02_Msg : Inport  Port=71
  C_LB_Batt2_CellVoltage02_Timeout : Inport  Port=72
  C_LB_Batt2_CellTemperature_Msg : Inport  Port=73
  C_LB_Batt2_CellTemperature_Timeout : Inport  Port=74
  C_LB_Batt2_InsulationMonitor_Msg : Inport  Port=75
  C_LB_Batt2_InsulationMonitor_Timeout : Inport  Port=76
  C_LB_Batt2_Status01_Msg : Inport  Port=77
  C_LB_Batt2_Status01_Timeout : Inport  Port=78
  C_LB_Batt2_Status02_Msg : Inport  Port=79
  C_LB_Batt2_Status02_Timeout : Inport  Port=80
  C_LB_Batt2_Status03_Msg : Inport  Port=81
  C_LB_Batt2_Status03_Timeout : Inport  Port=82
  C_LB_Batt3_CellVoltage01_Msg : Inport  Port=83
  C_LB_Batt3_CellVoltage01_Timeout : Inport  Port=84
  C_LB_Batt3_CellVoltage02_Msg : Inport  Port=85
  C_LB_Batt3_CellVoltage02_Timeout : Inport  Port=86
  C_LB_Batt3_CellTemperature_Msg : Inport  Port=87
  C_LB_Batt3_CellTemperature_Timeout : Inport  Port=88
  C_LB_Batt3_InsulationMonitor_Msg : Inport  Port=89
  C_LB_Batt3_InsulationMonitor_Timeout : Inport  Port=90
  C_LB_Batt3_Status01_Msg : Inport  Port=91
  C_LB_Batt3_Status01_Timeout : Inport  Port=92
  C_LB_Batt3_Status02_Msg : Inport  Port=93
  C_LB_Batt3_Status02_Timeout : Inport  Port=94
  C_LB_Batt3_Status03_Msg : Inport  Port=95
  C_LB_Batt3_Status03_Timeout : Inport  Port=96
  C_UDC_Msg1 : Inport  Port=97
  C_UDC_Msg1_Timeout : Inport  Port=98
  Flow Logic : Subsystem
  Input Processing : Subsystem
  Input Translation : Subsystem
  Output Processing : Subsystem
  Output Translation : Subsystem
  CMSleep : Outport
  DO_KL15_BB1 : Outport  Port=2
  DO_KL15_BB2 : Outport  Port=3
  DO_KL15_BB3 : Outport  Port=4
  DO_REQ_MainHV_ON_MINUS : Outport  Port=5
  DO_REQ_MainHV_ON_PLUS : Outport  Port=6
  DO_REQ_MainHV_ON_Precharge : Outport  Port=7
  DO_REQ_DC_ON_MINUS : Outport  Port=8
  DO_REQ_DC_ON_PLUS : Outport  Port=9
  DO_boKL15_IMD_BB1 : Outport  Port=10
  DO_boKL15_IMD_BB2 : Outport  Port=11
  DO_boKL15_IMD_BB3 : Outport  Port=12
  DO_CabinAlarm : Outport  Port=13
  DO_boEMSRET_BDU1 : Outport  Port=14  OutDataTypeStr=boolean
  DO_boEMSRET_BDU2 : Outport  Port=15  OutDataTypeStr=boolean
  DO_boEMSRET_BB1_1 : Outport  Port=16  OutDataTypeStr=boolean
  DO_boEMSRET_BB1_2 : Outport  Port=17  OutDataTypeStr=boolean
  DO_boEMSRET_BB2_1 : Outport  Port=18  OutDataTypeStr=boolean
  DO_boEMSRET_BB2_2 : Outport  Port=19  OutDataTypeStr=boolean
  DO_boEMSRET_BB3_1 : Outport  Port=20  OutDataTypeStr=boolean
  DO_boEMSRET_BB3_2 : Outport  Port=21  OutDataTypeStr=boolean
  DO_HVIL_Supply : Outport  Port=22  OutDataTypeStr=boolean
  DO_boResetButton_LED : Outport  Port=23  OutDataTypeStr=boolean
  BMS_Control_Batt1 : Outport  Port=24
  BMS_Control_Batt2 : Outport  Port=25
  BMS_Control_Batt3 : Outport  Port=26
  OP_LiBa_OperationRequest_Batt1 : Outport  Port=27
  OP_LiBa_OperationRequest_Batt2 : Outport  Port=28
  OP_LiBa_OperationRequest_Batt3 : Outport  Port=29
  OP_ChiefMaster_IP_Msg1 : Outport  Port=30
  OP_ChiefMaster_OP_Msg2 : Outport  Port=31
  OP_ChiefMaster_SS1_Msg3 : Outport  Port=32
  OP_ChiefMaster_SS2_Msg4 : Outport  Port=33
  OP_ChiefMaster_Calc_Msg5 : Outport  Port=34
  OP_ChiefMaster_BDU_Msg6 : Outport  Port=35
  OP_ChiefMaster_Battery1_Msg7 : Outport  Port=36
  OP_ChiefMaster_Battery1_Msg8 : Outport  Port=37
  OP_ChiefMaster_Battery1_Msg9 : Outport  Port=38
  OP_ChiefMaster_Battery2_Msg10 : Outport  Port=39
  OP_ChiefMaster_Battery2_Msg11 : Outport  Port=40
  OP_ChiefMaster_Battery2_Msg12 : Outport  Port=41
  OP_ChiefMaster_Battery3_Msg13 : Outport  Port=42
  OP_ChiefMaster_Battery3_Msg14 : Outport  Port=43
  OP_ChiefMaster_Battery3_Msg15 : Outport  Port=44
  wires:
  Input Translation/1(IT_Databus) -> Flow Logic/1(IT_Databus)
  C_LB_Batt1_InsulationMonitor_Msg/1 -> Input Processing/61(C_LB_Batt1_InsulationMonitor_Msg)
  C_LB_Batt1_CellVoltage02_Msg/1 -> Input Processing/57(C_LB_Batt1_CellVoltage02_Msg)
  Output Processing/6(DO_REQ_MainHV_ON_PLUS) -> DO_REQ_MainHV_ON_PLUS/1
  Output Processing/3(DO_KL15_BB2) -> DO_KL15_BB2/1
  Output Processing/7(DO_REQ_MainHV_ON_Precharge) -> DO_REQ_MainHV_ON_Precharge/1
  C_LB_Batt1_CellTemperature_Timeout/1 -> Input Processing/60(C_LB_Batt1_CellTemperature_Timeout)
  C_LB_Batt1_CellVoltage01_Timeout/1 -> Input Processing/56(C_LB_Batt1_CellVoltage01_Timeout)
  C_LB_BMS_Status02_Msg/1 -> Input Processing/65(C_LB_Batt1_Status02_Msg)
  Output Processing/24(OP_Actia_Control_Batt1) -> BMS_Control_Batt1/1
  C_LB_Batt1_Status03_Timeout/1 -> Input Processing/68(C_LB_Batt1_Status03_Timeout)
  C_LB_Batt1_Status01_Timeout/1 -> Input Processing/64(C_LB_Batt1_Status01_Timeout)
  C_LB_Batt1_Status01_Msg/1 -> Input Processing/63(C_LB_Batt1_Status01_Msg)
  C_LB_Batt1_CellTemperature_Msg/1 -> Input Processing/59(C_LB_Batt1_CellTemperature_Msg)
  C_LB_Batt1_CellVoltage01_Msg/1 -> Input Processing/55(C_LB_Batt1_CellVoltage01_Msg)
  Output Processing/2(DO_KL15_BB1) -> DO_KL15_BB1/1
  C_LB_Batt1_InsulationMonitor_Timeout/1 -> Input Processing/62(C_LB_Batt1_InsulationMonitor_Timeout)
  C_LB_Batt1_CellVoltage02_Timeout/1 -> Input Processing/58(C_LB_Batt1_CellVoltage02_Timeout)
  C_LB_Batt1_Status02_Timeout/1 -> Input Processing/66(C_LB_Batt1_Status02_Timeout)
  Input Processing/1(IP_Databus) -> Input Translation/1(IP_Databus)
  C_UDC_Msg1/1 -> Input Processing/97(C_UDC_Msg1_299)
  C_LB_Batt1_Status03_Msg/1 -> Input Processing/67(C_LB_Batt1_Status03_Msg)
  C_UDC_Msg1_Timeout/1 -> Input Processing/98(C_UDC_Msg1_299_Timeout)
  Output Processing/1(CMSleep) -> CMSleep/1
  Output Processing/4(DO_KL15_BB3) -> DO_KL15_BB3/1
  Output Processing/5(DO_REQ_MainHV_ON_MINUS) -> DO_REQ_MainHV_ON_MINUS/1
  Output Processing/25(OP_Actia_Control_Batt2) -> BMS_Control_Batt2/1
  Output Processing/26(OP_Actia_Control_Batt3) -> BMS_Control_Batt3/1
  C_LB_Batt3_Status02_Timeout/1 -> Input Processing/94(C_LB_Batt3_Status02_Timeout)
  C_LB_Batt3_CellVoltage01_Timeout/1 -> Input Processing/84(C_LB_Batt3_CellVoltage01_Timeout)
  C_LB_Batt3_CellVoltage02_Msg/1 -> Input Processing/85(C_LB_Batt3_CellVoltage02_Msg)
  C_LB_Batt3_Status03_Timeout/1 -> Input Processing/96(C_LB_Batt3_Status03_Timeout)
  C_LB_Batt3_Status03_Msg/1 -> Input Processing/95(C_LB_Batt3_Status03_Msg)
  C_LB_Batt2_Status01_Msg/1 -> Input Processing/77(C_LB_Batt2_Status01_Msg)
  C_LB_Batt2_Status01_Timeout/1 -> Input Processing/78(C_LB_Batt2_Status01_Timeout)
  C_LB_Batt3_Status02_Msg/1 -> Input Processing/93(C_LB_Batt3_Status02_Msg)
  C_LB_Batt2_InsulationMonitor_Timeout/1 -> Input Processing/76(C_LB_Batt2_InsulationMonitor_Timeout)
  C_LB_Batt2_InsulationMonitor_Msg/1 -> Input Processing/75(C_LB_Batt2_InsulationMonitor_Msg)
  C_LB_Batt2_CellTemperature_Msg/1 -> Input Processing/73(C_LB_Batt2_CellTemperature_Msg)
  C_LB_Batt2_CellVoltage02_Msg/1 -> Input Processing/71(C_LB_Batt2_CellVoltage02_Msg)
  C_LB_Batt2_CellVoltage02_Timeout/1 -> Input Processing/72(C_LB_Batt2_CellVoltage02_Timeout)
  C_LB_Batt2_CellTemperature_Timeout/1 -> Input Processing/74(C_LB_Batt2_CellTemperature_Timeout)
  C_LB_Batt3_CellVoltage02_Timeout/1 -> Input Processing/86(C_LB_Batt3_CellVoltage02_Timeout)
  C_LB_Batt3_CellTemperature_Msg/1 -> Input Processing/87(C_LB_Batt3_CellTemperature_Msg)
  C_LB_Batt3_CellTemperature_Timeout/1 -> Input Processing/88(C_LB_Batt3_CellTemperature_Timeout)
  C_LB_Batt3_CellVoltage01_Msg/1 -> Input Processing/83(C_LB_Batt3_CellVoltage01_Msg)
  C_LB_Batt3_InsulationMonitor_Msg/1 -> Input Processing/89(C_LB_Batt3_InsulationMonitor_Msg)
  C_LB_Batt3_InsulationMonitor_Timeout/1 -> Input Processing/90(C_LB_Batt3_InsulationMonitor_Timeout)
  C_LB_Batt2_Status03_Msg/1 -> Input Processing/81(C_LB_Batt2_Status03_Msg)
  C_LB_Batt2_Status02_Msg/1 -> Input Processing/79(C_LB_Batt2_Status02_Msg)
  C_LB_Batt2_Status02_Timeout/1 -> Input Processing/80(C_LB_Batt2_Status02_Timeout)
  C_LB_Batt3_Status01_Timeout/1 -> Input Processing/92(C_LB_Batt3_Status01_Timeout)
  C_LB_Batt2_Status03_Timeout/1 -> Input Processing/82(C_LB_Batt2_Status03_Timeout)
  C_LB_Batt2_CellVoltage01_Timeout/1 -> Input Processing/70(C_LB_Batt2_CellVoltage01_Timeout)
  C_LB_Batt3_Status01_Msg/1 -> Input Processing/91(C_LB_Batt3_Status01_Msg2)
  C_LB_Batt2_CellVoltage01_Msg/1 -> Input Processing/69(C_LB_Batt2_CellVoltage01_Msg)
  Output Processing/29(OP_LiBa_Control_Batt3) -> OP_LiBa_OperationRequest_Batt3/1
  Output Processing/27(OP_LiBa_Control_Batt1) -> OP_LiBa_OperationRequest_Batt1/1
  Output Processing/28(OP_LiBa_Control_Batt2) -> OP_LiBa_OperationRequest_Batt2/1
  Flow Logic/1(FL_Databus) -> Input Translation/2(IMD_Req_Databus), Output Translation/1(FL_Databus)
  DI_Proximity_BB1/1 -> Input Processing/11(DI_Proximity_BB1)
  AI_HVIL_Component/1 -> Input Processing/3(AI_HVIL_Component)
  AI_HVIL_BDU/1 -> Input Processing/2(AI_HVIL_BDU)
  AI_EmergencyButton_NO/1 -> Input Processing/9(AI_EmergencyButton_NO)
  AI_HVIL_Battery/1 -> Input Processing/4(AI_HVIL_Battery)
  DI_Proximity_BB3/1 -> Input Processing/13(DI_Proximity_BB3)
  AI_DCHV_Plus_FB/1 -> Input Processing/14(AI_DCHV_Plus_FB)
  AI_KL15/1 -> Input Processing/1(AI_KL15)
  AI_MainHV_Minus_FB/1 -> Input Processing/7(AI_MainHV_Minus_FB)
  DI_Proximity_BB2/1 -> Input Processing/12(DI_Proximity_BB2)
  AI_EmergencyButton_NC/1 -> Input Processing/8(AI_EmergencyButton_NC)
  AI_DCHV_Minus_FB/1 -> Input Processing/15(AI_DCHV_Minus_FB)
  DI_ResetButton_LED_NO/1 -> Input Processing/10(DI_ResetButton_LED_NO)
  AI_MainHV_Plus_FB/1 -> Input Processing/6(AI_MainHV_Plus_FB)
  C_Actia_Batt2_ADS_3/1 -> Input Processing/41(C_Actia_Batt2_ADS_3)
  C_Actia_Batt2_ADS_3_Timeout/1 -> Input Processing/42(C_Actia_Batt2_ADS_3_Timeout)
  C_Actia_Batt1_Error/1 -> Input Processing/21(C_Actia_Batt1_Error)
  C_Actia_Batt2_ADS_8_Timeout/1 -> Input Processing/36(C_Actia_Batt2_ADS_8_Timeout)
  C_Actia_Batt2_ADS_1_Timeout/1 -> Input Processing/40(C_Actia_Batt2_ADS_1_Timeout)
  C_Actia_Batt2_ADS_1/1 -> Input Processing/39(C_Actia_Batt2_ADS_1)
  C_Actia_Batt2_MyStatus/1 -> Input Processing/31(C_Actia_Batt2_MyStatus)
  C_Actia_Batt1_MyStatus/1 -> Input Processing/19(C_Actia_Batt1_MyStatus)
  C_Actia_Batt3_MyStatus/1 -> Input Processing/43(C_Actia_Batt3_MyStatus)
  C_Actia_Batt3_ADS_8_Timeout/1 -> Input Processing/48(C_Actia_Batt3_ADS_8_Timeout)
  C_Actia_Batt1_ADS_8/1 -> Input Processing/23(C_Actia_Batt1_ADS_8)
  C_Actia_Batt1_ADS_3/1 -> Input Processing/29(C_Actia_Batt1_ADS_3)
  C_Actia_Batt1_Error_Timeout/1 -> Input Processing/22(C_Actia_Batt1_Error_Timeout)
  C_Actia_Batt3_ADS_8/1 -> Input Processing/47(C_Actia_Batt3_ADS_8)
  C_Actia_Batt1_ADS_8_Timeout/1 -> Input Processing/24(C_Actia_Batt1_ADS_8_Timeout)
  C_Actia_Batt3_Error_Timeout/1 -> Input Processing/46(C_Actia_Batt3_Error_Timeout)
  C_Actia_Batt2_ADS_8/1 -> Input Processing/35(C_Actia_Batt2_ADS_8)
  C_Actia_Batt2_Error_Timeout/1 -> Input Processing/34(C_Actia_Batt2_Error_Timeout)
  C_Actia_Batt3_ADS_1/1 -> Input Processing/51(C_Actia_Batt3_ADS_1)
  C_Actia_Batt1_MyStatus_Timeout/1 -> Input Processing/20(C_Actia_Batt1_MyStatus_Timeout)
  C_Actia_Batt2_Error/1 -> Input Processing/33(C_Actia_Batt2_Error)
  C_Actia_Batt1_ADS_3_Timeout/1 -> Input Processing/30(C_Actia_Batt1_ADS_3_Timeout)
  C_Actia_Batt1_ADS_1_Timeout/1 -> Input Processing/28(C_Actia_Batt1_ADS_1_Timeout)
  C_Actia_Batt3_ADS_3_Timeout/1 -> Input Processing/54(C_Actia_Batt3_ADS_3_Timeout)
  C_Actia_Batt3_ADS_3/1 -> Input Processing/53(C_Actia_Batt3_ADS_3)
  C_Actia_Batt2_MyStatus_Timeout/1 -> Input Processing/32(C_Actia_Batt2_MyStatus_Timeout)
  C_Actia_Batt1_ADS_1/1 -> Input Processing/27(C_Actia_Batt1_ADS_1)
  C_Actia_Batt3_ADS_1_Timeout/1 -> Input Processing/52(C_Actia_Batt3_ADS_1_Timeout)
  C_Actia_Batt3_MyStatus_Timeout/1 -> Input Processing/44(C_Actia_Batt3_MyStatus_Timeout)
  C_Actia_Batt3_Error/1 -> Input Processing/45(C_Actia_Batt3_Error)
  Output Translation/1(OT_Databus) -> Output Processing/1(OT_Databus)
  Output Processing/30(OP_ChiefMaster_IP_Msg1) -> OP_ChiefMaster_IP_Msg1/1
  Output Processing/31(OP_ChiefMaster_OP_Msg2) -> OP_ChiefMaster_OP_Msg2/1
  Output Processing/32(OP_ChiefMaster_SS1_Msg3) -> OP_ChiefMaster_SS1_Msg3/1
  Output Processing/34(OP_ChiefMaster_Calc_Msg5) -> OP_ChiefMaster_Calc_Msg5/1
  Output Processing/33(OP_ChiefMaster_SS2_Msg4) -> OP_ChiefMaster_SS2_Msg4/1
  Output Processing/43(OP_ChiefMaster_Battery3_Msg14) -> OP_ChiefMaster_Battery3_Msg14/1
  Output Processing/42(OP_ChiefMaster_Battery3_Msg13) -> OP_ChiefMaster_Battery3_Msg13/1
  Output Processing/40(OP_ChiefMaster_Battery2_Msg11) -> OP_ChiefMaster_Battery2_Msg11/1
  Output Processing/39(OP_ChiefMaster_Battery2_Msg10) -> OP_ChiefMaster_Battery2_Msg10/1
  Output Processing/37(OP_ChiefMaster_Battery1_Msg8) -> OP_ChiefMaster_Battery1_Msg8/1
  Output Processing/36(OP_ChiefMaster_Battery1_Msg7) -> OP_ChiefMaster_Battery1_Msg7/1
  Output Processing/35(OP_ChiefMaster_BDU_Msg6) -> OP_ChiefMaster_BDU_Msg6/1
  Output Processing/8(DO_REQ_DC_ON_MINUS) -> DO_REQ_DC_ON_MINUS/1
  Output Processing/9(DO_REQ_DC_ON_PLUS) -> DO_REQ_DC_ON_PLUS/1
  C_Actia_Batt1_ADS_0_Timeout/1 -> Input Processing/26(C_Actia_Batt1_ADS_0_Timeout)
  C_Actia_Batt1_ADS_0/1 -> Input Processing/25(C_Actia_Batt1_ADS_0)
  C_Actia_Batt2_ADS_0/1 -> Input Processing/37(C_Actia_Batt2_ADS_0)
  C_Actia_Batt2_ADS_0_Timeout/1 -> Input Processing/38(C_Actia_Batt2_ADS_0_Timeout)
  C_Actia_Batt3_ADS_0_Timeout/1 -> Input Processing/50(C_Actia_Batt3_ADS_0_Timeout)
  C_Actia_Batt3_ADS_0/1 -> Input Processing/49(C_Actia_Batt3_ADS_0)
  Output Processing/38(OP_ChiefMaster_Battery1_Msg9) -> OP_ChiefMaster_Battery1_Msg9/1
  Output Processing/44(OP_ChiefMaster_Battery3_Msg15) -> OP_ChiefMaster_Battery3_Msg15/1
  Output Processing/41(OP_ChiefMaster_Battery2_Msg12) -> OP_ChiefMaster_Battery2_Msg12/1
  DI_HVIL_Overrule/1 -> Input Processing/5(DI_HVIL_Overrule)
  Output Processing/10(DO_boKL15_IMD_BB1) -> DO_boKL15_IMD_BB1/1
  Output Processing/11(DO_boKL15_IMD_BB2) -> DO_boKL15_IMD_BB2/1
  Output Processing/12(DO_boKL15_IMD_BB3) -> DO_boKL15_IMD_BB3/1
  DI_IMD_FB_BB1/1 -> Input Processing/16(DI_IMD_FB_BB1)
  DI_IMD_FB_BB2/1 -> Input Processing/17(DI_IMD_FB_BB2)
  DI_IMD_FB_BB3/1 -> Input Processing/18(DI_IMD_FB_BB3)
  Output Processing/13(DO_CabinAlarm) -> DO_CabinAlarm/1
  Output Processing/14(DO_boEMSRET_BDU1) -> DO_boEMSRET_BDU1/1
  Output Processing/15(DO_boEMSRET_BDU2) -> DO_boEMSRET_BDU2/1
  Output Processing/16(DO_boEMSRET_BB1_1) -> DO_boEMSRET_BB1_1/1
  Output Processing/17(DO_boEMSRET_BB1_2) -> DO_boEMSRET_BB1_2/1
  Output Processing/18(DO_boEMSRET_BB2_1) -> DO_boEMSRET_BB2_1/1
  Output Processing/21(DO_boEMSRET_BB3_2) -> DO_boEMSRET_BB3_2/1
  Output Processing/20(DO_boEMSRET_BB3_1) -> DO_boEMSRET_BB3_1/1
  Output Processing/19(DO_boEMSRET_BB2_2) -> DO_boEMSRET_BB2_2/1
  Output Processing/22(DO_HVIL_Supply) -> DO_HVIL_Supply/1
  Output Processing/23(DO_boResetButton_LED) -> DO_boResetButton_LED/1

== system ChiefMaster_TTC580/ChiefMaster/Flow Logic ==
  IT_Databus : Inport
  BDU Control : Subsystem
  Battery HVControl : Subsystem
  Bus Creator1 : BusCreator  Inputs=7
  IMD Control : Subsystem
  KL15 : Subsystem
  Reset : Subsystem
  System Status : Subsystem
  FL_Databus : Outport
  wires:
  Reset/1(FL_ResetReq_Databus) -> Bus Creator1/6, [ResetReq_DataBus]
  Battery HVControl/1(FL_BatteryBox_HVControl_Databus) -> Bus Creator1/3, [BattHVControl]
  BDU Control/1(FL_BDUControl_Databus) -> [BDUControl_Databus], Bus Creator1/4
  System Status/1(FL_SystemStatus_Databus) -> [Status_Databus], Bus Creator1/5
  Bus Creator1/1 -> FL_Databus/1  "FL_Databus"
  KL15/1(FL_KL15_Databus) -> [KL15_DataBus], Bus Creator1/1
  [KL15_DataBus] -> Battery HVControl/2(FL_KL15_Databus)
  [KL15_DataBus] -> BDU Control/2(FL_KL15_Databus)
  [KL15_DataBus] -> Reset/1(FL_KL15_Databus)
  [BDUControl_Databus] -> System Status/1(FL_BDUControl_Databus)
  [KL15_DataBus] -> System Status/2(FL_KL15_Databus)
  [BDUControl_Databus] -> Battery HVControl/4(FL_BDUControl_Databus)
  [BattHVControl] -> BDU Control/1(FL_BatteryBox_HVControl_Databus)
  [BattHVControl] -> System Status/5(FL_BatteryBox_HVControl_Databus)
  [BattHVControl] -> KL15/2(FL_BatteryBox_HVControl_Databus)
  [ResetReq_DataBus] -> Battery HVControl/1(Reset_Req_Databus)
  [ResetReq_DataBus] -> KL15/3(Reset_Req_Databus)
  [BattHVControl] -> Reset/3(FL_BatteryBox_HVControl_Databus)
  [Status_Databus] -> BDU Control/4(FL_SystemStatus_Databus)
  [Status_Databus] -> Battery HVControl/5(FL_SystemStatus_Databus)
  [Status_Databus] -> IMD Control/2(FL_SystemStatus_Databus)
  IT_Databus/1 -> KL15/1(IT_Databus), IMD Control/1(IT_Databus), Battery HVControl/3(IT_Databus), Bus Creator1/7, Reset/2(IT_Databus), System Status/3(IT_Databus), BDU Control/3(IT_Databus)
  IMD Control/1(FL_IMD_Control_Databus) -> [IMD_Databus], Bus Creator1/2
  [IMD_Databus] -> System Status/4(FL_IMD_Control_Databus)
